simulink model "Lab5_Lag"  (R2016a)
settings: Solver=VariableStepAuto  StartTime=0.0  StopTime=60.0  RelTol=1e-3
settings Model: Creator=jordan  LastModifiedBy=jordan

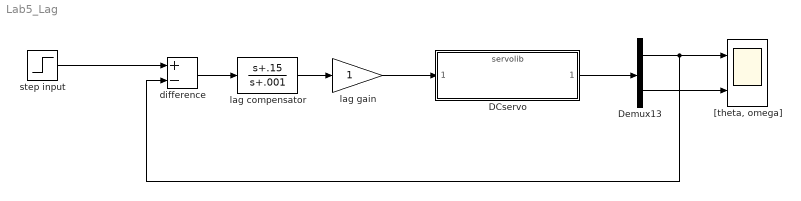
== system Lab5_Lag ==
  DCservo : ModelReference  ModelNameDialog=servolib.slx  SimulationMode=Normal  ModelReferenceVersion=1.18
  Demux13 : Demux  Outputs=2
  "[theta, omega]" : Scope  NumInputPorts=2
  difference : Sum  Inputs=+-
  lag compensator : TransferFcn  Numerator=[1 .15]  Denominator=[1 .001]
  lag gain : Gain
  step input : Step  SampleTime=0
  wires:
  Demux13/2 -> "[theta, omega]"/2
  difference/1 -> lag compensator/1
  Demux13/1 -> difference/2, "[theta, omega]"/1
  step input/1 -> difference/1
  lag compensator/1 -> lag gain/1
  lag gain/1 -> DCservo/1
  DCservo/1 -> Demux13/1
